simulink model "esn"  (R2024a)
settings: Solver=VariableStepAuto  StartTime=0.0  StopTime=stoptime  RelTol=1e-3
values from neighbouring files (symbols this model uses):
  esn = ESN_trainbysim(Nr, 'sizeinput', sizeinput, 'nodenuminput', 3, 'sizeoutput', sizeoutput,          'timeConst', timeConstant, 'spectralRadius', SR, 'inputScaling', 1, 'connectivity', 0.5, 'biasScaling', 0,          'regularization', 1e-1, 'delaylen', 0.1, 'timestep', 0.01, 'normmethod', normmethod, 'ifxnorm', ifxnorm, 'sizereadout', Nr + sizeinput + 1)    [stmpcevaluation.m]
settings Model: Creator=fy264  LastModifiedBy=fy264
settings DebuggingCC: AlgebraicLoopMsg=none  ArtificialAlgebraicLoopMsg=none
settings RTWCC: GPUComputeCapability=3.5

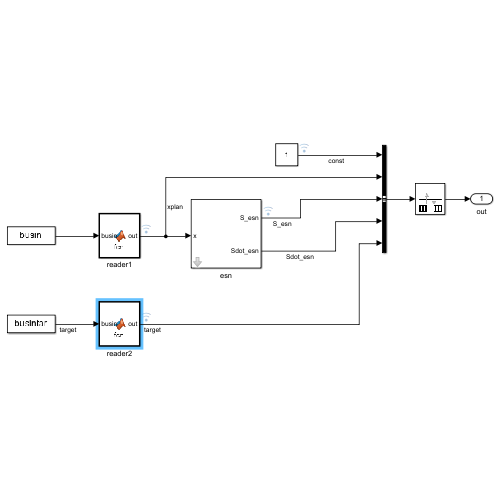
[thumbnail: Simulink's stored preview of the top-level diagram]
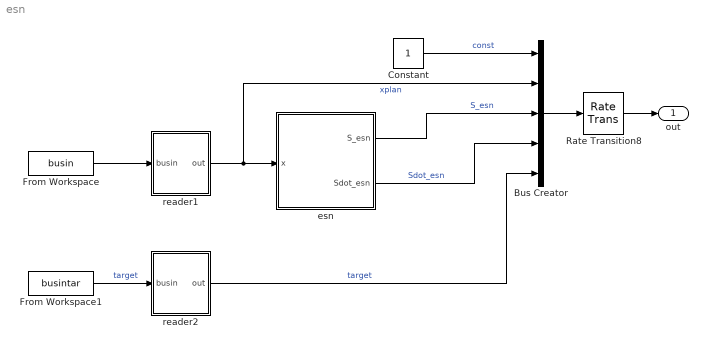
== system esn ==
  Bus Creator : BusCreator  Inputs=5
  Constant : Constant
  From Workspace : FromWorkspace  VariableName=busin  OutDataTypeStr=Bus: SinusoidBus  Interpolate=off  OutputAfterFinalValue=Holding final value
  From Workspace1 : FromWorkspace  VariableName=busintar  OutDataTypeStr=Bus: SinusoidBustar  Interpolate=off  OutputAfterFinalValue=Holding final value
  Rate Transition8 : RateTransition  OutPortSampleTime=esn.timestep
  esn : Subsystem  mask{Nr=esn.Nr, sizeinput=esn.sizeinput, nodenuminput=esn.nodenuminput, Win=esn.Win, Wr=esn.Wr, Wb=esn.Wb, tau=esn.tau, timestep=esn.timestep, ini_S=esn.initialstate}
  reader1 : MATLAB Function  TreatAsAtomicUnit=on
  reader2 : MATLAB Function  TreatAsAtomicUnit=on
  out : Outport
  wires:
  esn/1(S_esn) -> Bus Creator/3  "S_esn"
  From Workspace/1 -> reader1/1(busin)
  Bus Creator/1 -> Rate Transition8/1
  Rate Transition8/1 -> out/1
  Constant/1 -> Bus Creator/1  "const"
  esn/2(Sdot_esn) -> Bus Creator/4  "Sdot_esn"
  From Workspace1/1 -> reader2/1(busin)  "target"
  reader1/1(out) -> Bus Creator/2, esn/1(x)  "xplan"
  reader2/1(out) -> Bus Creator/5  "target"

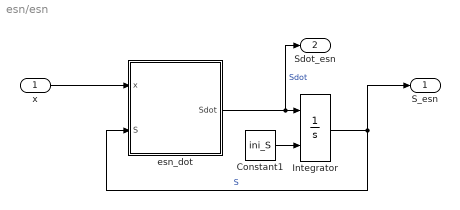
== system esn/esn ==
  x : Inport
  Constant1 : Constant  Value=ini_S  VectorParams1D=off
  Integrator : Integrator  InitialConditionSource=external
  esn_dot : MATLAB Function  TreatAsAtomicUnit=on
  S_esn : Outport
  Sdot_esn : Outport  Port=2
  wires:
  esn_dot/1(Sdot) -> Sdot_esn/1, Integrator/1  "Sdot"
  Integrator/1 -> S_esn/1, esn_dot/2(S)  "S"
  Constant1/1 -> Integrator/2
  x/1 -> esn_dot/1(x)

== matlab function esn/reader2 ==
  data: busin input; out output
function out = fcn(busin)

buscell = struct2cell(busin);
out = zeros(20,1);
for i = 1:20
    out(i,1) = buscell{i}(1);
end

end

== matlab function esn/esn_dot ==
  data: x input; Sdot output; S input; Nr parameter; sizeinput parameter; nodenuminput parameter; Win parameter; Wr parameter; Wb parameter; tau parameter
function Sdot = fcn(x, S, Nr, sizeinput, nodenuminput, Win, Wr, Wb, tau)

u = zeros(Nr, 1);
for j = 1:sizeinput
    u(j:(j+nodenuminput-1)) = x(j,1);
end

Sdot = (-S + tanh(Win.*u + Wr*S + Wb))/tau;

== matlab function esn/reader1 ==
  data: busin input; out output
function out = fcn(busin)

buscell = struct2cell(busin);

out = buscell{1}(1);

end
